simulink model "cubli_ZYX"  (R2016a)
settings: Solver=FixedStepAuto  StartTime=0.0  StopTime=10  FixedStep=0.001  RelTol=1e-3
values from neighbouring files (symbols this model uses):
  a = 0.15    [init.m]
  M = 2.5    [init.m]    (also in skew.m = [0 -z y)
  m = 0.204    [init.m]
  s = size(delta_i)    [accessibility_test.m]    (also in observability_test.m = size(delta_i,1))
  state0 = get_equilibrium(0, -pi/4, pi/2, f, state)    [init.m]
undefined symbols (not defined in the file or in its folder): X, Y, Z
libraries: sm_lib x15, nesl_utility x9
settings Model: Creator=giulio  LastModifiedBy=giulio
settings OptimizationCC: BlockReduction=off  DefaultParameterBehavior=Inlined  BufferReuse=off
settings GRTTargetCC: GeneratePreprocessorConditionals=Use local settings
settings SimscapeCC: SimscapeLogType=all  SimscapeLogDataHistory=10000

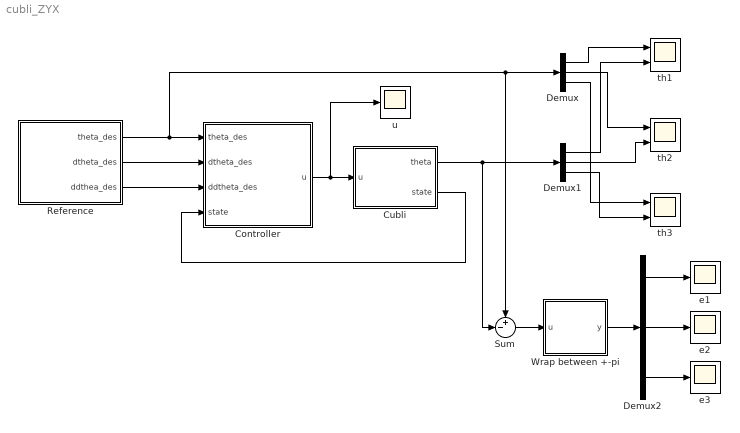
== system cubli_ZYX ==
  Controller : Subsystem
  Cubli : Subsystem
  Demux : Demux  Outputs=3
  Demux1 : Demux  Outputs=3
  Demux2 : Demux  Outputs=3
  Reference : Subsystem  mask{theta=170.0, final_time=5}
      mask prompts: final_time "Final time"
  Sum : Sum  Inputs=+-|
  Wrap between +-pi : MATLAB Function  TreatAsAtomicUnit=on
  e1 : Scope
  e2 : Scope
  e3 : Scope
  th1 : Scope  NumInputPorts=2
  th2 : Scope  NumInputPorts=2
  th3 : Scope  NumInputPorts=2
  u : Scope
  wires:
  Cubli/1(theta) -> Demux1/1, Sum/2
  Cubli/2(state) -> Controller/4(state)
  Demux/1 -> th1/1
  Demux1/1 -> th1/2
  Demux/2 -> th2/1
  Demux1/2 -> th2/2
  Demux/3 -> th3/1
  Demux1/3 -> th3/2
  Wrap between +-pi/1(y) -> Demux2/1
  Sum/1 -> Wrap between +-pi/1(u)
  Demux2/3 -> e3/1
  Demux2/1 -> e1/1
  Demux2/2 -> e2/1
  Controller/1(u) -> u/1, Cubli/1(u)
  Reference/1(theta_des) -> Controller/1(theta_des), Demux/1, Sum/1
  Reference/2(dtheta_des) -> Controller/2(dtheta_des)
  Reference/3("ddthea_des ") -> Controller/3(ddtheta_des)

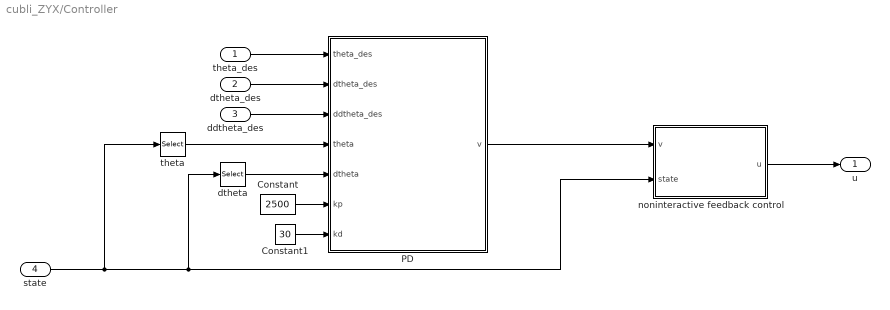
== system cubli_ZYX/Controller ==
  theta_des : Inport
  dtheta_des : Inport  Port=2
  ddtheta_des : Inport  Port=3
  state : Inport  Port=4
  Constant : Constant  Value=2500
  Constant1 : Constant  Value=30
  PD : MATLAB Function  TreatAsAtomicUnit=on
  dtheta : Selector  InputPortWidth=9  IndexOptions=Index vector (dialog)  Indices=[4 5 6]  OutputSizes=1
  noninteractive feedback control : MATLAB Function  TreatAsAtomicUnit=on
  theta : Selector  InputPortWidth=9  IndexOptions=Index vector (dialog)  Indices=[1 2 3]  OutputSizes=1
  u : Outport
  wires:
  theta_des/1 -> PD/1(theta_des)
  state/1 -> theta/1, noninteractive feedback control/2(state), dtheta/1
  PD/1(v) -> noninteractive feedback control/1(v)
  dtheta/1 -> PD/5(dtheta)
  dtheta_des/1 -> PD/2(dtheta_des)
  ddtheta_des/1 -> PD/3(ddtheta_des)
  theta/1 -> PD/4(theta)
  Constant/1 -> PD/6(kp)
  Constant1/1 -> PD/7(kd)
  noninteractive feedback control/1(u) -> u/1

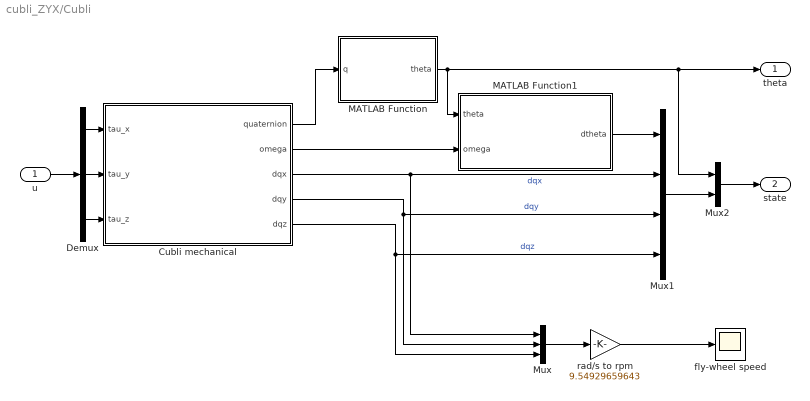
== system cubli_ZYX/Cubli ==
  u : Inport
  "Cubli mechanical " : Subsystem
  Demux : Demux  Outputs=3
  MATLAB Function : MATLAB Function  TreatAsAtomicUnit=on
  MATLAB Function1 : MATLAB Function  TreatAsAtomicUnit=on
  Mux : Mux  Inputs=3
  Mux1 : Mux
  Mux2 : Mux  Inputs=2
  fly-wheel speed : Scope
  rad/s to rpm : Gain  Gain=9.54929659643
  theta : Outport
  state : Outport  Port=2
  wires:
  Mux1/1 -> Mux2/2
  Demux/3 -> "Cubli mechanical "/3(tau_z)
  Demux/2 -> "Cubli mechanical "/2(tau_y)
  Demux/1 -> "Cubli mechanical "/1(tau_x)
  u/1 -> Demux/1
  Mux2/1 -> state/1
  "Cubli mechanical "/4(dqy) -> Mux/2, Mux1/3  "dqy"
  "Cubli mechanical "/5(dqz) -> Mux/3, Mux1/4  "dqz"
  "Cubli mechanical "/3(dqx) -> Mux/1, Mux1/2  "dqx"
  Mux/1 -> rad/s to rpm/1
  rad/s to rpm/1 -> fly-wheel speed/1
  "Cubli mechanical "/1(quaternion) -> MATLAB Function/1(q)
  MATLAB Function/1(theta) -> MATLAB Function1/1(theta), theta/1, Mux2/1
  MATLAB Function1/1(dtheta) -> Mux1/1
  "Cubli mechanical "/2(omega) -> MATLAB Function1/2(omega)

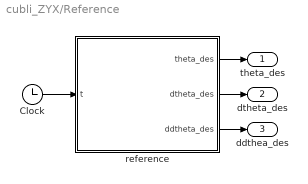
== system cubli_ZYX/Reference ==
  Clock : Clock
  reference : MATLAB Function  TreatAsAtomicUnit=on
  theta_des : Outport
  dtheta_des : Outport  Port=2
  "ddthea_des " : Outport  Port=3
  wires:
  reference/1(theta_des) -> theta_des/1
  reference/2(dtheta_des) -> dtheta_des/1
  reference/3(ddtheta_des) -> "ddthea_des "/1
  Clock/1 -> reference/1(t)

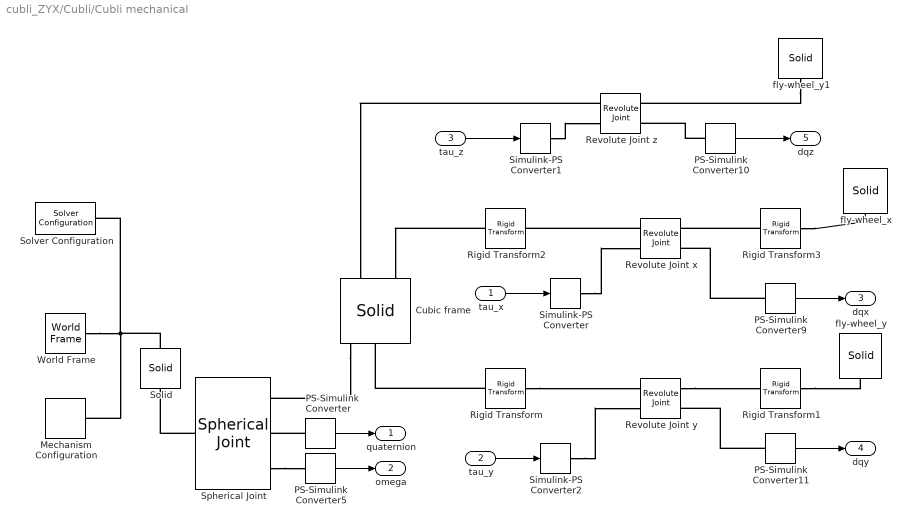
== system cubli_ZYX/Cubli/Cubli mechanical  ==
  tau_x : Inport
  tau_y : Inport  Port=2
  tau_z : Inport  Port=3
  Cubic frame : sm_lib/Body Elements/Solid  InertiaType=CalculateFromGeometry  Mass=M  MassUnits=kg  CenterOfMass=[0 0 0]  CenterOfMassUnits=m  MomentsOfInertia=[1 1 1]  MomentsOfInertiaUnits=kg*m^2  ProductsOfInertia=[0 0 0]  ProductsOfInertiaUnits=kg*m^2  DensityBased=off  Density=1000  DensityUnits=kg/(m^3)  DoExposeReferenceFrame=off  SerializedFrames=<Frames><Frame><Id>Frame1</Id><Value><Name>Oc</Name><Origin><Source>GeometricFeature</Source><FeatureName>-x -y -z point</FeatureName></Origin><PrimaryAxis><DefinedDirection>+Z</DefinedDirection><Source>ReferenceFrame</Source><SourceDirection>+Z</SourceDirection><FeatureName></FeatureName></PrimaryAxis><SecondaryAxis><DefinedDirection>+X</DefinedDirection><Source>ReferenceFrame</Source><SourceDirection>+X</SourceDirection><FeatureName></FeatureName></SecondaryAxis></Value></Frame><Frame><Id>Frame2</Id><Value><Name>Oz</Name><Origin><Source>GeometricFeature</Source><FeatureName>-z surface</FeatureName></Origin><PrimaryAxis><DefinedDirection>+Z</DefinedDirection><Source>ReferenceFrame</Source><SourceDirection>+Z</SourceDirection><FeatureName></FeatureName></PrimaryAxis><SecondaryAxis><DefinedDirection>+X</DefinedDirection><Source>ReferenceFrame</Source><SourceDirection>+X</SourceDirection><FeatureName></FeatureName></SecondaryAxis></Value></Frame><Frame><Id>Frame3</Id><Value><Name>Oy</Name><Origin><Source>GeometricFeature</Source><FeatureName>-y surface</FeatureName></Origin><PrimaryAxis><DefinedDirection>+Z</DefinedDirection><Source>ReferenceFrame</Source><SourceDirection>+Z</SourceDirection><FeatureName></FeatureName></PrimaryAxis><SecondaryAxis><DefinedDirection>+X</DefinedDirection><Source>ReferenceFrame</Source><SourceDirection>+X</SourceDirection><FeatureName></FeatureName></SecondaryAxis></Value></Frame><Frame><Id>Frame4</Id><Value><Name>Ox</Name><Origin><Source>GeometricFeature</Source><FeatureName>-x surface</FeatureName></Origin><PrimaryAxis><DefinedDirection>+Z</DefinedDirection><Source>ReferenceFrame</Source><SourceDirection>+Z</SourceDirection><FeatureName></FeatureName></PrimaryAxis><SecondaryAxis><DefinedDirection>+X</DefinedDirection><Source>ReferenceFrame</Source><SourceDirection>+X</SourceDirection><FeatureName></FeatureName></SecondaryAxis></Value></Frame><Frame><Id>Frame5</Id><Value><Name>Op</Name><Origin><Source>GeometricFeature</Source><FeatureName>+x +y +z point</FeatureName></Origin><PrimaryAxis><DefinedDirection>+Z</DefinedDirection><Source>ReferenceFrame</Source><SourceDirection>+Z</SourceDirection><FeatureName></FeatureName></PrimaryAxis><SecondaryAxis><DefinedDirection>+X</DefinedDirection><Source>ReferenceFrame</Source><SourceDirection>+X</SourceDirection><FeatureName></FeatureName></SecondaryAxis></Value></Frame></Frames>  GraphicType=FromGeometry  MarkerShape=Sphere  MarkerSize=10  GraphicVisPropType=SimpleVisualProperties  GraphicDiffuseColor=[0.5 0.5 0.5]  GraphicSpecularColor=[0.5 0.5 0.5 1.0]  GraphicAmbientColor=[0.15 0.15 0.15 1.0]  GraphicEmissiveColor=[0.0 0.0 0.0 1.0]  GraphicShininess=75  GraphicOpacity=0.9  GeometryShape=Brick  RectangleSize=[1 1]  RectangleSizeUnits=m  BrickDimensions=[a a a]  BrickDimensionUnits=m  CylinderRadius=1  CylinderRadiusUnits=m  CylinderLength=1  CylinderLengthUnits=m  SphereRadius=1  SphereRadiusUnits=m  EllipsoidRadii=[1 1 1]  EllipsoidRadiiUnits=m  ExtrusionCrossSection=[1 1; -1 1; -1 -1; 1 -1]  ExtrusionCrossSectionUnits=m  ExtrusionLength=1  ExtrusionLengthUnits=m  PolygonNumSides=3  PolygonOuterRadius=1  PolygonOuterRadiusUnits=m  ExtGeomFileType=STEP  ExtGeomFileUnits=m  RevolutionCrossSection=[1 1; 1 -1; 2 -1; 2 1]  RevolutionCrossSectionUnits=m  RevolutionExtent=Full  RevolutionAngle=180  RevolutionAngleUnits=deg
  Mechanism Configuration : sm_lib/Utilities/Mechanism Configuration  UniformGravity=Constant  GravityVector=[0 0 -9.81]  GravityUnits=m/s^2  LinearizationDelta=0.001
  PS-Simulink Converter{,5,9..11} (5 alike) : nesl_utility/PS-Simulink Converter  PhysicalDomain=network_engine_domain  SubClassName=ps_output  LeftPortType=input  RightPortType=output  PseudoPeriodic=off  Frequencies=[]  Unit=1  AffineConversion=off
  Revolute Joint x : sm_lib/Joints/Revolute Joint  SenseConstraintForce=off  SenseConstraintForceX=off  SenseConstraintForceY=off  SenseConstraintForceZ=off  SenseConstraintTorque=off  SenseConstraintTorqueX=off  SenseConstraintTorqueY=off  SenseConstraintTorqueZ=off  SenseTotalForce=off  SenseTotalForceX=off  SenseTotalForceY=off  SenseTotalForceZ=off  SenseTotalTorque=off  SenseTotalTorqueX=off  SenseTotalTorqueY=off  SenseTotalTorqueZ=off  CompositeWrenchDir=FollowerOnBase  CompositeWrenchFrame=BaseFrame  EquilibriumPosition=0  EquilibriumPositionUnits=deg  SpringStiffness=0  SpringStiffnessUnits=N*m/deg  DampingCoefficient=0  DampingCoefficientUnits=N*m/(rad/s)  TorqueActuationMode=InputTorque  MotionActuationMode=ComputedMotion  SensePosition=off  SenseVelocity=on  SenseAcceleration=off  SenseTorqueForce=off  PositionTargetSpecify=off  PositionTargetPriority=High  PositionTargetValue=0  PositionTargetValueUnits=deg  VelocityTargetSpecify=off  VelocityTargetPriority=High  VelocityTargetValue=0  VelocityTargetValueUnits=deg/s
  Revolute Joint y : sm_lib/Joints/Revolute Joint  SenseConstraintForce=off  SenseConstraintForceX=off  SenseConstraintForceY=off  SenseConstraintForceZ=off  SenseConstraintTorque=off  SenseConstraintTorqueX=off  SenseConstraintTorqueY=off  SenseConstraintTorqueZ=off  SenseTotalForce=off  SenseTotalForceX=off  SenseTotalForceY=off  SenseTotalForceZ=off  SenseTotalTorque=off  SenseTotalTorqueX=off  SenseTotalTorqueY=off  SenseTotalTorqueZ=off  CompositeWrenchDir=FollowerOnBase  CompositeWrenchFrame=BaseFrame  EquilibriumPosition=0  EquilibriumPositionUnits=deg  SpringStiffness=0  SpringStiffnessUnits=N*m/deg  DampingCoefficient=0  DampingCoefficientUnits=N*m/(rad/s)  TorqueActuationMode=InputTorque  MotionActuationMode=ComputedMotion  SensePosition=off  SenseVelocity=on  SenseAcceleration=off  SenseTorqueForce=off  PositionTargetSpecify=off  PositionTargetPriority=High  PositionTargetValue=0  PositionTargetValueUnits=deg  VelocityTargetSpecify=off  VelocityTargetPriority=High  VelocityTargetValue=0  VelocityTargetValueUnits=deg/s
  Revolute Joint z : sm_lib/Joints/Revolute Joint  SenseConstraintForce=off  SenseConstraintForceX=off  SenseConstraintForceY=off  SenseConstraintForceZ=off  SenseConstraintTorque=off  SenseConstraintTorqueX=off  SenseConstraintTorqueY=off  SenseConstraintTorqueZ=off  SenseTotalForce=off  SenseTotalForceX=off  SenseTotalForceY=off  SenseTotalForceZ=off  SenseTotalTorque=off  SenseTotalTorqueX=off  SenseTotalTorqueY=off  SenseTotalTorqueZ=off  CompositeWrenchDir=FollowerOnBase  CompositeWrenchFrame=BaseFrame  EquilibriumPosition=0  EquilibriumPositionUnits=deg  SpringStiffness=0  SpringStiffnessUnits=N*m/deg  DampingCoefficient=0  DampingCoefficientUnits=N*m/(rad/s)  TorqueActuationMode=InputTorque  MotionActuationMode=ComputedMotion  SensePosition=off  SenseVelocity=on  SenseAcceleration=off  SenseTorqueForce=off  PositionTargetSpecify=off  PositionTargetPriority=High  PositionTargetValue=0  PositionTargetValueUnits=deg  VelocityTargetSpecify=off  VelocityTargetPriority=High  VelocityTargetValue=1/6  VelocityTargetValueUnits=rev/s
  Rigid Transform : sm_lib/Frames and Transforms/Rigid Transform  TranslationMethod=None  TranslationLengthUnit=m  TranslationStandardAxis=+Z  TranslationStandardOffset=0  TranslationCartesianOffset=[0 0 0]  TranslationROffset=0  TranslationROffsetUnits=m  TranslationZOffset=0  TranslationZOffsetUnits=m  TranslationThetaOffset=0  TranslationThetaOffsetUnits=deg  RotationMethod=RotationSequence  RotationAngleUnits=deg  RotationStandardAxis=+Z  RotationAngle=0.0  RotationArbitraryAxis=[0 0 1]  FollAlignAxisA=+X  BaseAlignAxisA=+Y  FollAlignAxisB=+Y  BaseAlignAxisB=+Z  RotationSequenceAxes=FollowerAxes  RotationSequence=XYX  RotationSequenceAngles=[-90 0 0]  RotationSequenceAnglesUnits=deg  RotationMatrix=[1 0 0; 0 1 0; 0 0 1]
  Rigid Transform1 : sm_lib/Frames and Transforms/Rigid Transform  TranslationMethod=None  TranslationLengthUnit=m  TranslationStandardAxis=+Z  TranslationStandardOffset=0  TranslationCartesianOffset=[0 0 0]  TranslationROffset=0  TranslationROffsetUnits=m  TranslationZOffset=0  TranslationZOffsetUnits=m  TranslationThetaOffset=0  TranslationThetaOffsetUnits=deg  RotationMethod=RotationSequence  RotationAngleUnits=deg  RotationStandardAxis=+Z  RotationAngle=0.0  RotationArbitraryAxis=[0 0 1]  FollAlignAxisA=+X  BaseAlignAxisA=+Y  FollAlignAxisB=+Y  BaseAlignAxisB=+Z  RotationSequenceAxes=FollowerAxes  RotationSequence=XYX  RotationSequenceAngles=[90 0 0]  RotationSequenceAnglesUnits=deg  RotationMatrix=[1 0 0; 0 1 0; 0 0 1]
  Rigid Transform2 : sm_lib/Frames and Transforms/Rigid Transform  TranslationMethod=None  TranslationLengthUnit=m  TranslationStandardAxis=+Z  TranslationStandardOffset=0  TranslationCartesianOffset=[0 0 0]  TranslationROffset=0  TranslationROffsetUnits=m  TranslationZOffset=0  TranslationZOffsetUnits=m  TranslationThetaOffset=0  TranslationThetaOffsetUnits=deg  RotationMethod=RotationSequence  RotationAngleUnits=deg  RotationStandardAxis=+Z  RotationAngle=0.0  RotationArbitraryAxis=[0 0 1]  FollAlignAxisA=+X  BaseAlignAxisA=+Y  FollAlignAxisB=+Y  BaseAlignAxisB=+Z  RotationSequenceAxes=FollowerAxes  RotationSequence=XYX  RotationSequenceAngles=[0 90 0]  RotationSequenceAnglesUnits=deg  RotationMatrix=[1 0 0; 0 1 0; 0 0 1]
  Rigid Transform3 : sm_lib/Frames and Transforms/Rigid Transform  TranslationMethod=None  TranslationLengthUnit=m  TranslationStandardAxis=+Z  TranslationStandardOffset=0  TranslationCartesianOffset=[0 0 0]  TranslationROffset=0  TranslationROffsetUnits=m  TranslationZOffset=0  TranslationZOffsetUnits=m  TranslationThetaOffset=0  TranslationThetaOffsetUnits=deg  RotationMethod=RotationSequence  RotationAngleUnits=deg  RotationStandardAxis=+Z  RotationAngle=0.0  RotationArbitraryAxis=[0 0 1]  FollAlignAxisA=+X  BaseAlignAxisA=+Y  FollAlignAxisB=+Y  BaseAlignAxisB=+Z  RotationSequenceAxes=FollowerAxes  RotationSequence=XYX  RotationSequenceAngles=[0 -90 0]  RotationSequenceAnglesUnits=deg  RotationMatrix=[1 0 0; 0 1 0; 0 0 1]
  Simulink-PS Converter : nesl_utility/Simulink-PS Converter  PhysicalDomain=network_engine_domain  SubClassName=ps_input  LeftPortType=input  RightPortType=output  PseudoPeriodic=off  Frequencies=[]  NoiseDistribution=none  NoiseParameters=[]  Unit=1  AffineConversion=off  InputFiltering=off  SimscapeFilterOrder=1  InputFilterTimeConstant=0.001  UdotUserProvided=1
  Simulink-PS Converter1 : nesl_utility/Simulink-PS Converter  PhysicalDomain=network_engine_domain  SubClassName=ps_input  LeftPortType=input  RightPortType=output  PseudoPeriodic=off  Frequencies=[]  NoiseDistribution=none  NoiseParameters=[]  Unit=1  AffineConversion=off  InputFiltering=off  SimscapeFilterOrder=1  InputFilterTimeConstant=0.001  UdotUserProvided=1
  Simulink-PS Converter2 : nesl_utility/Simulink-PS Converter  PhysicalDomain=network_engine_domain  SubClassName=ps_input  LeftPortType=input  RightPortType=output  PseudoPeriodic=off  Frequencies=[]  NoiseDistribution=none  NoiseParameters=[]  Unit=1  AffineConversion=off  InputFiltering=off  SimscapeFilterOrder=1  InputFilterTimeConstant=0.001  UdotUserProvided=1
  Solid : sm_lib/Body Elements/Solid  InertiaType=CalculateFromGeometry  Mass=10^5  MassUnits=kg  CenterOfMass=[0 0 0]  CenterOfMassUnits=m  MomentsOfInertia=[1 1 1]  MomentsOfInertiaUnits=kg*m^2  ProductsOfInertia=[0 0 0]  ProductsOfInertiaUnits=kg*m^2  DensityBased=off  Density=1000  DensityUnits=kg/(m^3)  DoExposeReferenceFrame=on  SerializedFrames=<Frames><Frame><Id>Frame1</Id><Value><Name>Os</Name><Origin><Source>GeometricFeature</Source><FeatureName>+z surface</FeatureName></Origin><PrimaryAxis><DefinedDirection>+Z</DefinedDirection><Source>ReferenceFrame</Source><SourceDirection>+Z</SourceDirection><FeatureName></FeatureName></PrimaryAxis><SecondaryAxis><DefinedDirection>+X</DefinedDirection><Source>ReferenceFrame</Source><SourceDirection>+X</SourceDirection><FeatureName></FeatureName></SecondaryAxis></Value></Frame></Frames>  GraphicType=FromGeometry  MarkerShape=Sphere  MarkerSize=10  GraphicVisPropType=SimpleVisualProperties  GraphicDiffuseColor=[1.0 1.0 1.0]  GraphicSpecularColor=[0.5 0.5 0.5 1.0]  GraphicAmbientColor=[1 0.15 0.15 1.0]  GraphicEmissiveColor=[0.0 0.0 0.0 1.0]  GraphicShininess=75  GraphicOpacity=1.0  GeometryShape=Brick  RectangleSize=[1 1]  RectangleSizeUnits=m  BrickDimensions=[1 1 0.01]  BrickDimensionUnits=m  CylinderRadius=1  CylinderRadiusUnits=m  CylinderLength=1  CylinderLengthUnits=m  SphereRadius=1  SphereRadiusUnits=m  EllipsoidRadii=[1 1 1]  EllipsoidRadiiUnits=m  ExtrusionCrossSection=[1 1; -1 1; -1 -1; 1 -1]  ExtrusionCrossSectionUnits=m  ExtrusionLength=1  ExtrusionLengthUnits=m  PolygonNumSides=3  PolygonOuterRadius=1  PolygonOuterRadiusUnits=m  ExtGeomFileType=STEP  ExtGeomFileUnits=m  RevolutionCrossSection=[1 1; 1 -1; 2 -1; 2 1]  RevolutionCrossSectionUnits=m  RevolutionExtent=Full  RevolutionAngle=180  RevolutionAngleUnits=deg
  Solver Configuration : nesl_utility/Solver Configuration  PhysicalDomain=network_engine_domain  SubClassName=solver  LeftPortType=input  RightPortType=generic  Accelerate=off  Tones=[]  Harmonics=[]  SimulateNoise=off  Profile=off  UseLocalSampling=off  EnableSwitchedLinearOptims=on  FrequencyDomain=off  UseCCode=off  RelTol=0.001  AbsTol=1e-06  MinStep=1e-09  ToWorkspace=off  RevertToSquareIcSolve=off  NumHomotopyIterations=100  PhasorMode=off  PhasorModeNumHarmonics=1  OverrideAbsTol=off  DoDC=on  ResidualTolerance=1e-09  UseLocalSolver=off  LocalSolverChoice=NE_TRAPEZOIDAL_ADVANCER  LocalSolverSampleTime=0.001  DoFixedCost=off  MaxNonlinIter=3  MaxModeIter=2  LinearAlgebra=Full  DelaysMemoryBudget=1024  AutomaticFiltering=on  FilteringTimeConstant=0.001
  Spherical Joint : sm_lib/Joints/Spherical Joint  SenseConstraintForce=off  SenseConstraintForceX=off  SenseConstraintForceY=off  SenseConstraintForceZ=off  SenseConstraintTorque=off  SenseConstraintTorqueX=off  SenseConstraintTorqueY=off  SenseConstraintTorqueZ=off  SenseTotalForce=off  SenseTotalForceX=off  SenseTotalForceY=off  SenseTotalForceZ=off  SenseTotalTorque=off  SenseTotalTorqueX=off  SenseTotalTorqueY=off  SenseTotalTorqueZ=off  CompositeWrenchDir=FollowerOnBase  CompositeWrenchFrame=BaseFrame  DefPosRotationMethod=None  DefPosRotationAngleUnits=deg  DefPosRotationStandardAxis=+Z  DefPosRotationAngle=0.0  DefPosRotationArbitraryAxis=[0 0 1]  DefPosFollAlignAxisA=+X  DefPosBaseAlignAxisA=+Y  DefPosFollAlignAxisB=+Y  DefPosBaseAlignAxisB=+Z  DefPosRotationSequenceAxes=FollowerAxes  DefPosRotationSequence=XYX  DefPosRotationSequenceAngles=[0 0 0]  DefPosRotationSequenceAnglesUnits=deg  DefPosRotationMatrix=[1 0 0; 0 1 0; 0 0 1]  EqPosRotationMethod=None  EqPosRotationAngleUnits=deg  EqPosRotationStandardAxis=+Z  EqPosRotationAngle=0.0  EqPosRotationArbitraryAxis=[0 0 1]  EqPosFollAlignAxisA=+X  EqPosBaseAlignAxisA=+Y  EqPosFollAlignAxisB=+Y  EqPosBaseAlignAxisB=+Z  EqPosRotationSequenceAxes=FollowerAxes  EqPosRotationSequence=XYX  EqPosRotationSequenceAngles=[0 0 0]  EqPosRotationSequenceAnglesUnits=deg  EqPosRotationMatrix=[1 0 0; 0 1 0; 0 0 1]  SpringStiffness=0  SpringStiffnessUnits=N*m/deg  DampingCoefficient=0  DampingCoefficientUnits=N*m/(deg/s)  ActuateTorqueX=off  ActuateTorqueY=off  ActuateTorqueZ=off  ActuateTorque=off  TorqueActuationMode=NoTorque  MotionActuationMode=ComputedMotion  ActuationFrame=BaseFrame  SensePosition=on  SenseVelocityX=off  SenseVelocityY=off  SenseVelocityZ=off  SenseVelocity=on  SenseAccelerationX=off  SenseAccelerationY=off  SenseAccelerationZ=off  SenseAcceleration=off  SenseTorqueX=off  SenseTorqueY=off  SenseTorqueZ=off  SenseTorqueForce=off  SensingFrame=FollowerFrame  PositionTargetRotationMethod=RotationSequence  PositionTargetRotationAngleUnits=deg  PositionTargetRotationStandardAxis=+Z  PositionTargetRotationAngle=0.0  PositionTargetRotationArbitraryAxis=[0 0 1]  PositionTargetFollAlignAxisA=+X  PositionTargetBaseAlignAxisA=+Y  PositionTargetFollAlignAxisB=+Y  PositionTargetBaseAlignAxisB=+Z  PositionTargetRotationSequenceAxes=FollowerAxes  PositionTargetRotationSequence=ZYX  PositionTargetRotationSequenceAngles=[state0(1) state0(2) state0(3)]  PositionTargetRotationSequenceAnglesUnits=rad  PositionTargetRotationMatrix=[1 0 0; 0 1 0; 0 0 1]  PositionTargetSpecify=on  PositionTargetPriority=High  VelocityTargetValue=[0 0 0]  VelocityTargetValueUnits=deg/s  VelocityTargetSpecify=off  VelocityTargetPriority=High  VelocityTargetInFollowerFrame=on
  World Frame : sm_lib/Frames and Transforms/World Frame
  fly-wheel_x : sm_lib/Body Elements/Solid  InertiaType=CalculateFromGeometry  Mass=m  MassUnits=kg  CenterOfMass=[0 0 0]  CenterOfMassUnits=m  MomentsOfInertia=[1 1 1]  MomentsOfInertiaUnits=kg*m^2  ProductsOfInertia=[0 0 0]  ProductsOfInertiaUnits=kg*m^2  DensityBased=off  Density=1000  DensityUnits=kg/(m^3)  DoExposeReferenceFrame=off  SerializedFrames=<Frames><Frame><Id>Frame1</Id><Value><Name>Ox</Name><Origin><Source>ReferenceFrame</Source><FeatureName></FeatureName></Origin><PrimaryAxis><DefinedDirection>-X</DefinedDirection><Source>ReferenceFrame</Source><SourceDirection>+Z</SourceDirection><FeatureName></FeatureName></PrimaryAxis><SecondaryAxis><DefinedDirection>+Y</DefinedDirection><Source>ReferenceFrame</Source><SourceDirection>+X</SourceDirection><FeatureName></FeatureName></SecondaryAxis></Value></Frame></Frames>  GraphicType=FromGeometry  MarkerShape=Sphere  MarkerSize=10  GraphicVisPropType=SimpleVisualProperties  GraphicDiffuseColor=[1.0 0.0 0.0]  GraphicSpecularColor=[0.5 0.5 0.5 1.0]  GraphicAmbientColor=[0.15 0.15 0.15 1.0]  GraphicEmissiveColor=[0.0 0.0 0.0 1.0]  GraphicShininess=75  GraphicOpacity=1  GeometryShape=Cylinder  RectangleSize=[1 1]  RectangleSizeUnits=m  BrickDimensions=[a a a]  BrickDimensionUnits=m  CylinderRadius=r  CylinderRadiusUnits=m  CylinderLength=h  CylinderLengthUnits=m  SphereRadius=1  SphereRadiusUnits=m  EllipsoidRadii=[1 1 1]  EllipsoidRadiiUnits=m  ExtrusionCrossSection=[1 1; -1 1; -1 -1; 1 -1]  ExtrusionCrossSectionUnits=m  ExtrusionLength=1  ExtrusionLengthUnits=m  PolygonNumSides=3  PolygonOuterRadius=1  PolygonOuterRadiusUnits=m  ExtGeomFileType=STEP  ExtGeomFileUnits=m  RevolutionCrossSection=[1 1; 1 -1; 2 -1; 2 1]  RevolutionCrossSectionUnits=m  RevolutionExtent=Full  RevolutionAngle=180  RevolutionAngleUnits=deg
  fly-wheel_y : sm_lib/Body Elements/Solid  InertiaType=CalculateFromGeometry  Mass=m  MassUnits=kg  CenterOfMass=[0 0 0]  CenterOfMassUnits=m  MomentsOfInertia=[1 1 1]  MomentsOfInertiaUnits=kg*m^2  ProductsOfInertia=[0 0 0]  ProductsOfInertiaUnits=kg*m^2  DensityBased=off  Density=1000  DensityUnits=kg/(m^3)  DoExposeReferenceFrame=off  SerializedFrames=<Frames><Frame><Id>Frame1</Id><Value><Name>Oy</Name><Origin><Source>ReferenceFrame</Source><FeatureName></FeatureName></Origin><PrimaryAxis><DefinedDirection>+Y</DefinedDirection><Source>ReferenceFrame</Source><SourceDirection>+Z</SourceDirection><FeatureName></FeatureName></PrimaryAxis><SecondaryAxis><DefinedDirection>+X</DefinedDirection><Source>ReferenceFrame</Source><SourceDirection>+X</SourceDirection><FeatureName></FeatureName></SecondaryAxis></Value></Frame></Frames>  GraphicType=FromGeometry  MarkerShape=Sphere  MarkerSize=10  GraphicVisPropType=SimpleVisualProperties  GraphicDiffuseColor=[0.0 0.8 0.0]  GraphicSpecularColor=[0.5 0.5 0.5 1.0]  GraphicAmbientColor=[0.15 0.15 0.15 1.0]  GraphicEmissiveColor=[0.0 0.0 0.0 1.0]  GraphicShininess=75  GraphicOpacity=1  GeometryShape=Cylinder  RectangleSize=[1 1]  RectangleSizeUnits=m  BrickDimensions=[a a a]  BrickDimensionUnits=m  CylinderRadius=r  CylinderRadiusUnits=m  CylinderLength=h  CylinderLengthUnits=m  SphereRadius=1  SphereRadiusUnits=m  EllipsoidRadii=[1 1 1]  EllipsoidRadiiUnits=m  ExtrusionCrossSection=[1 1; -1 1; -1 -1; 1 -1]  ExtrusionCrossSectionUnits=m  ExtrusionLength=1  ExtrusionLengthUnits=m  PolygonNumSides=3  PolygonOuterRadius=1  PolygonOuterRadiusUnits=m  ExtGeomFileType=STEP  ExtGeomFileUnits=m  RevolutionCrossSection=[1 1; 1 -1; 2 -1; 2 1]  RevolutionCrossSectionUnits=m  RevolutionExtent=Full  RevolutionAngle=180  RevolutionAngleUnits=deg
  fly-wheel_y1 : sm_lib/Body Elements/Solid  InertiaType=CalculateFromGeometry  Mass=m  MassUnits=kg  CenterOfMass=[0 0 0]  CenterOfMassUnits=m  MomentsOfInertia=[1 1 1]  MomentsOfInertiaUnits=kg*m^2  ProductsOfInertia=[0 0 0]  ProductsOfInertiaUnits=kg*m^2  DensityBased=off  Density=1000  DensityUnits=kg/(m^3)  DoExposeReferenceFrame=off  SerializedFrames=<Frames><Frame><Id>Frame1</Id><Value><Name>Oz</Name><Origin><Source>ReferenceFrame</Source><FeatureName></FeatureName></Origin><PrimaryAxis><DefinedDirection>+Z</DefinedDirection><Source>ReferenceFrame</Source><SourceDirection>+Z</SourceDirection><FeatureName></FeatureName></PrimaryAxis><SecondaryAxis><DefinedDirection>+X</DefinedDirection><Source>ReferenceFrame</Source><SourceDirection>+X</SourceDirection><FeatureName></FeatureName></SecondaryAxis></Value></Frame></Frames>  GraphicType=FromGeometry  MarkerShape=Sphere  MarkerSize=10  GraphicVisPropType=SimpleVisualProperties  GraphicDiffuseColor=[0.0 0.0 1.0]  GraphicSpecularColor=[0.5 0.5 0.5 1.0]  GraphicAmbientColor=[0.15 0.15 0.15 1.0]  GraphicEmissiveColor=[0.0 0.0 0.0 1.0]  GraphicShininess=75  GraphicOpacity=1  GeometryShape=Cylinder  RectangleSize=[1 1]  RectangleSizeUnits=m  BrickDimensions=[a a a]  BrickDimensionUnits=m  CylinderRadius=r  CylinderRadiusUnits=m  CylinderLength=h  CylinderLengthUnits=m  SphereRadius=1  SphereRadiusUnits=m  EllipsoidRadii=[1 1 1]  EllipsoidRadiiUnits=m  ExtrusionCrossSection=[1 1; -1 1; -1 -1; 1 -1]  ExtrusionCrossSectionUnits=m  ExtrusionLength=1  ExtrusionLengthUnits=m  PolygonNumSides=3  PolygonOuterRadius=1  PolygonOuterRadiusUnits=m  ExtGeomFileType=STL  ExtGeomFileName=/home/xenvre/Downloads/flywheel/Flywheel.stl  ExtGeomFileUnits=cm  RevolutionCrossSection=[1 1; 1 -1; 2 -1; 2 1]  RevolutionCrossSectionUnits=m  RevolutionExtent=Full  RevolutionAngle=180  RevolutionAngleUnits=deg
  quaternion : Outport
  omega : Outport  Port=2
  dqx : Outport  Port=3
  dqy : Outport  Port=4
  dqz : Outport  Port=5
  wires:
  tau_y/1 -> Simulink-PS Converter2/1
  tau_z/1 -> Simulink-PS Converter1/1
  tau_x/1 -> Simulink-PS Converter/1
  PS-Simulink Converter/1 -> quaternion/1
  PS-Simulink Converter9/1 -> dqx/1
  PS-Simulink Converter10/1 -> dqz/1
  PS-Simulink Converter11/1 -> dqy/1
  PS-Simulink Converter5/1 -> omega/1
  connections:
  Rigid Transform3/LConn1 -- Revolute Joint x/RConn1
  fly-wheel_y1/LConn1 -- Revolute Joint z/RConn1
  Simulink-PS Converter2/RConn1 -- Revolute Joint y/LConn2
  Simulink-PS Converter/RConn1 -- Revolute Joint x/LConn2
  Rigid Transform1/RConn1 -- fly-wheel_y/LConn1
  Cubic frame/LConn1 -- Spherical Joint/RConn1
  World Frame/RConn1 -- Solid/RConn1 -- Solver Configuration/RConn1 -- Mechanism Configuration/RConn1
  Simulink-PS Converter1/RConn1 -- Revolute Joint z/LConn2
  Revolute Joint y/RConn1 -- Rigid Transform1/LConn1
  Revolute Joint x/LConn1 -- Rigid Transform2/RConn1
  Rigid Transform/RConn1 -- Revolute Joint y/LConn1
  PS-Simulink Converter/LConn1 -- Spherical Joint/RConn2
  PS-Simulink Converter9/LConn1 -- Revolute Joint x/RConn2
  PS-Simulink Converter10/LConn1 -- Revolute Joint z/RConn2
  PS-Simulink Converter11/LConn1 -- Revolute Joint y/RConn2
  Rigid Transform2/LConn1 -- Cubic frame/RConn2
  Revolute Joint z/LConn1 -- Cubic frame/RConn1
  Rigid Transform/LConn1 -- Cubic frame/LConn2
  Rigid Transform3/RConn1 -- fly-wheel_x/LConn1
  Spherical Joint/LConn1 -- Solid/LConn1
  Spherical Joint/RConn3 -- PS-Simulink Converter5/LConn1

== matlab function cubli_ZYX/Controller/PD ==
  data: theta_des input; dtheta_des input; ddtheta_des input; theta input; v output; dtheta input; kp input; kd input
function v = fcn(theta_des,dtheta_des,ddtheta_des, theta, dtheta, kp, kd)
coder.extrinsic('wrapToPi');

error = zeros(3,1);

%  wrap the angle bewteen -pi and +pi
error = wrapToPi(theta_des - theta);

Kp = kp * eye(3);
Kd = kd * eye(3);

v = Kp * error + Kd * (dtheta_des - dtheta) + ddtheta_des;

== matlab function cubli_ZYX/Controller/noninteractive feedback control ==
  data: v input; state input; u output
  function u = nic_fnc(v, state)

th1 = state(1);
th2 = state(2);
th3 = state(3);

th1dot = state(4);
th2dot = state(5);
th3dot = state(6);
qxdot = state(7);
qydot = state(8);
qzdot = state(9);


A = [                                                                   -(1123197656438253912603716965936891166720000*2^(1/2)*sin(th3 + pi/4))/(50688073959935957106266099682798465939237*cos(th2)),                                                    -(11529215046068469760000*(97421867139278569472*cos(th3) + 173808361171031714041*sin(th3)))/(50688073959935957106266099682798465939237*cos(th2)),                                                    -(11529215046068469760000*(173808361171031714041*cos(th3) + 97421867139278569472*sin(th3)))/(50688073959935957106266099682798465939237*cos(th2))
                                                                                   -(1123197656438253912603716965936891166720000*2^(1/2)*cos(th3 + pi/4))/50688073959935957106266099682798465939237, (1123197656438253912603716965936891166720000*sin(th3))/50688073959935957106266099682798465939237 - (2003873972745561633640040521298775900160000*cos(th3))/50688073959935957106266099682798465939237, (2003873972745561633640040521298775900160000*sin(th3))/50688073959935957106266099682798465939237 - (1123197656438253912603716965936891166720000*cos(th3))/50688073959935957106266099682798465939237
 -(11529215046068469760000*(173808361171031714041*cos(th2) + 97421867139278569472*cos(th3)*sin(th2) + 97421867139278569472*sin(th2)*sin(th3)))/(50688073959935957106266099682798465939237*cos(th2)),  -(11529215046068469760000*(97421867139278569472*cos(th2) + 97421867139278569472*cos(th3)*sin(th2) + 173808361171031714041*sin(th2)*sin(th3)))/(50688073959935957106266099682798465939237*cos(th2)),  -(11529215046068469760000*(97421867139278569472*cos(th2) + 173808361171031714041*cos(th3)*sin(th2) + 97421867139278569472*sin(th2)*sin(th3)))/(50688073959935957106266099682798465939237*cos(th2))];
 

b = [                                                                                                                                                                                                                                                                                                                                                                                                                                                                                                                                                                                                                                                                                                                                                                                                                                                                                                                                                                                                                                                                                                                                                                                                                                                                                                                                                                                                (37208574363983751213784670214039629987840*th1dot^2*cos(th3) - 37208574363983751213784670214039629987840*th2dot^2*cos(th3) + 37208574363983751213784670214039629987840*th3dot^2*cos(th3) - 37208574363983751213784670214039629987840*th1dot^2*sin(th3) + 37208574363983751213784670214039629987840*th2dot^2*sin(th3) - 37208574363983751213784670214039629987840*th3dot^2*sin(th3) - 5234057499985498930356104062315637394898944*cos(th3)*sin(th2) + 5234057499985498930356104062315637394898944*sin(th2)*sin(th3) + 1419410730694772925795933922925238500000*qxdot*th2dot - 795598339977096578581794905915392000000*qydot*th2dot + 140800205444266547517405832452217960942325*th2dot*th3dot + 18604287181991875606892335107019814993920*th1dot^2*sin(2*th2) + 795598339977096578581794905915392000000*qxdot*th1dot*cos(th2) - 1419410730694772925795933922925238500000*qydot*th3dot*cos(th3) - 795598339977096578581794905915392000000*qzdot*th1dot*cos(th2) + 795598339977096578581794905915392000000*qzdot*th3dot*cos(th3) - 37208574363983751213784670214039629987840*th1dot*th3dot*cos(th2) - 795598339977096578581794905915392000000*qydot*th3dot*sin(th3) + 1419410730694772925795933922925238500000*qzdot*th3dot*sin(th3) + 140800205444266547517405832452217960942325*th1dot*th2dot*sin(th2) - 37208574363983751213784670214039629987840*th1dot^2*cos(th2)^2*cos(th3) + 37208574363983751213784670214039629987840*th1dot^2*cos(th2)^2*sin(th3) + 795598339977096578581794905915392000000*qydot*th2dot*cos(th3)^2 - 795598339977096578581794905915392000000*qzdot*th2dot*cos(th3)^2 + 795598339977096578581794905915392000000*qxdot*th2dot*sin(2*th3) - 397799169988548289290897452957696000000*qydot*th2dot*sin(2*th3) - 397799169988548289290897452957696000000*qzdot*th2dot*sin(2*th3) - 37208574363983751213784670214039629987840*th2dot*th3dot*sin(2*th3) + 1419410730694772925795933922925238500000*qydot*th1dot*cos(th3)*sin(th2) - 795598339977096578581794905915392000000*qzdot*th1dot*cos(th3)*sin(th2) - 37208574363983751213784670214039629987840*th1dot*th2dot*cos(th2)*sin(th3) - 74417148727967502427569340428079259975680*th1dot*th3dot*cos(th3)*sin(th2) + 795598339977096578581794905915392000000*qydot*th1dot*sin(th2)*sin(th3) - 1419410730694772925795933922925238500000*qzdot*th1dot*sin(th2)*sin(th3) + 74417148727967502427569340428079259975680*th1dot*th3dot*sin(th2)*sin(th3) - 74417148727967502427569340428079259975680*th1dot^2*cos(th2)*cos(th3)^2*sin(th2) - 1591196679954193157163589811830784000000*qxdot*th1dot*cos(th2)*cos(th3)^2 + 795598339977096578581794905915392000000*qydot*th1dot*cos(th2)*cos(th3)^2 + 795598339977096578581794905915392000000*qzdot*th1dot*cos(th2)*cos(th3)^2 + 74417148727967502427569340428079259975680*th1dot*th3dot*cos(th2)*cos(th3)^2 - 37208574363983751213784670214039629987840*th1dot*th2dot*cos(th2)*cos(th3) + 795598339977096578581794905915392000000*qydot*th1dot*cos(th2)*cos(th3)*sin(th3) - 795598339977096578581794905915392000000*qzdot*th1dot*cos(th2)*cos(th3)*sin(th3) + 74417148727967502427569340428079259975680*th1dot*th2dot*cos(th3)*sin(th2)*sin(th3))/(140800205444266547517405832452217960942325*cos(th2))
                                                                                                                                                                                                                                                                                                                                                                                                                                                                                                                                                                                             (68520719092170281189376*cos(th2))/1843260477247944264925 - (97421867139278569472*th1dot^2*cos(th3))/368652095449588852985 - (97421867139278569472*th3dot^2*cos(th3))/368652095449588852985 - (97421867139278569472*th1dot^2*sin(th3))/368652095449588852985 - (97421867139278569472*th3dot^2*sin(th3))/368652095449588852985 + (68520719092170281189376*cos(th3)*sin(th2))/1843260477247944264925 + (68520719092170281189376*sin(th2)*sin(th3))/1843260477247944264925 - (31823933599083863143271796236615680000*qxdot*th2dot)/5632008217770661900696233298088718437693 + (31823933599083863143271796236615680000*qydot*th2dot)/5632008217770661900696233298088718437693 + (97421867139278569472*th2dot*th3dot)/368652095449588852985 - (56776429227790917031837356917009540000*qxdot*th1dot*cos(th2))/5632008217770661900696233298088718437693 - (31823933599083863143271796236615680000*qydot*th3dot*cos(th3))/5632008217770661900696233298088718437693 + (31823933599083863143271796236615680000*qzdot*th1dot*cos(th2))/5632008217770661900696233298088718437693 + (56776429227790917031837356917009540000*qzdot*th3dot*cos(th3))/5632008217770661900696233298088718437693 - th1dot*th3dot*cos(th2) + (56776429227790917031837356917009540000*qydot*th3dot*sin(th3))/5632008217770661900696233298088718437693 - (31823933599083863143271796236615680000*qzdot*th3dot*sin(th3))/5632008217770661900696233298088718437693 - (97421867139278569472*th1dot*th2dot*sin(th2))/368652095449588852985 + (194843734278557138944*th1dot^2*cos(th2)^2*cos(th3))/368652095449588852985 + (194843734278557138944*th1dot^2*cos(th2)^2*sin(th3))/368652095449588852985 + (63647867198167726286543592473231360000*qxdot*th2dot*cos(th3)^2)/5632008217770661900696233298088718437693 - (31823933599083863143271796236615680000*qydot*th2dot*cos(th3)^2)/5632008217770661900696233298088718437693 - (31823933599083863143271796236615680000*qzdot*th2dot*cos(th3)^2)/5632008217770661900696233298088718437693 - (194843734278557138944*th2dot*th3dot*cos(th3)^2)/368652095449588852985 - (15911966799541931571635898118307840000*qydot*th2dot*sin(2*th3))/5632008217770661900696233298088718437693 + (15911966799541931571635898118307840000*qzdot*th2dot*sin(2*th3))/5632008217770661900696233298088718437693 + (31823933599083863143271796236615680000*qydot*th1dot*cos(th3)*sin(th2))/5632008217770661900696233298088718437693 - (56776429227790917031837356917009540000*qzdot*th1dot*cos(th3)*sin(th2))/5632008217770661900696233298088718437693 - (97421867139278569472*th1dot*th2dot*cos(th2)*sin(th3))/368652095449588852985 + (194843734278557138944*th1dot*th3dot*cos(th3)*sin(th2))/368652095449588852985 - (56776429227790917031837356917009540000*qydot*th1dot*sin(th2)*sin(th3))/5632008217770661900696233298088718437693 + (31823933599083863143271796236615680000*qzdot*th1dot*sin(th2)*sin(th3))/5632008217770661900696233298088718437693 + (194843734278557138944*th1dot*th3dot*sin(th2)*sin(th3))/368652095449588852985 + (31823933599083863143271796236615680000*qydot*th1dot*cos(th2)*cos(th3)^2)/5632008217770661900696233298088718437693 - (31823933599083863143271796236615680000*qzdot*th1dot*cos(th2)*cos(th3)^2)/5632008217770661900696233298088718437693 + (194843734278557138944*th1dot*th2dot*cos(th3)^2*sin(th2))/368652095449588852985 + (97421867139278569472*th1dot*th2dot*cos(th2)*cos(th3))/368652095449588852985 + (194843734278557138944*th1dot^2*cos(th2)*cos(th3)*sin(th2)*sin(th3))/368652095449588852985 + (63647867198167726286543592473231360000*qxdot*th1dot*cos(th2)*cos(th3)*sin(th3))/5632008217770661900696233298088718437693 - (31823933599083863143271796236615680000*qydot*th1dot*cos(th2)*cos(th3)*sin(th3))/5632008217770661900696233298088718437693 - (31823933599083863143271796236615680000*qzdot*th1dot*cos(th2)*cos(th3)*sin(th3))/5632008217770661900696233298088718437693 - (194843734278557138944*th1dot*th3dot*cos(th2)*cos(th3)*sin(th3))/368652095449588852985
 (5234057499985498930356104062315637394898944*sin(th3) - 5234057499985498930356104062315637394898944*cos(th3) + 37208574363983751213784670214039629987840*th1dot^2*cos(th2) - 37208574363983751213784670214039629987840*th2dot^2*cos(th2) + 140800205444266547517405832452217960942325*th1dot*th2dot - 37208574363983751213784670214039629987840*th1dot^2*sin(th2)*sin(th3) + 37208574363983751213784670214039629987840*th2dot^2*sin(th2)*sin(th3) - 37208574363983751213784670214039629987840*th3dot^2*sin(th2)*sin(th3) + 1419410730694772925795933922925238500000*qydot*th1dot*cos(th3) - 795598339977096578581794905915392000000*qydot*th3dot*cos(th2) - 795598339977096578581794905915392000000*qzdot*th1dot*cos(th3) + 795598339977096578581794905915392000000*qzdot*th3dot*cos(th2) - 74417148727967502427569340428079259975680*th1dot*th3dot*cos(th3) + 1419410730694772925795933922925238500000*qxdot*th2dot*sin(th2) + 795598339977096578581794905915392000000*qydot*th1dot*sin(th3) - 795598339977096578581794905915392000000*qydot*th2dot*sin(th2) - 1419410730694772925795933922925238500000*qzdot*th1dot*sin(th3) + 74417148727967502427569340428079259975680*th1dot*th3dot*sin(th3) + 140800205444266547517405832452217960942325*th2dot*th3dot*sin(th2) - 74417148727967502427569340428079259975680*th1dot^2*cos(th2)*cos(th3)^2 + 74417148727967502427569340428079259975680*th2dot^2*cos(th2)*cos(th3)^2 + 397799169988548289290897452957696000000*qxdot*th1dot*sin(2*th2) + 397799169988548289290897452957696000000*qydot*th1dot*sin(2*th2) - 795598339977096578581794905915392000000*qzdot*th1dot*sin(2*th2) + 37208574363983751213784670214039629987840*th1dot*th2dot*sin(2*th3) - 18604287181991875606892335107019814993920*th1dot*th3dot*sin(2*th2) + 37208574363983751213784670214039629987840*th1dot^2*cos(th3)*sin(th2) - 37208574363983751213784670214039629987840*th2dot^2*cos(th3)*sin(th2) + 37208574363983751213784670214039629987840*th3dot^2*cos(th3)*sin(th2) + 795598339977096578581794905915392000000*qxdot*th2dot*cos(th2)*sin(th3) - 1419410730694772925795933922925238500000*qydot*th2dot*cos(th2)*sin(th3) - 1419410730694772925795933922925238500000*qydot*th3dot*cos(th3)*sin(th2) + 795598339977096578581794905915392000000*qzdot*th3dot*cos(th3)*sin(th2) + 37208574363983751213784670214039629987840*th2dot*th3dot*cos(th2)*sin(th3) - 795598339977096578581794905915392000000*qydot*th3dot*sin(th2)*sin(th3) + 1419410730694772925795933922925238500000*qzdot*th3dot*sin(th2)*sin(th3) - 795598339977096578581794905915392000000*qxdot*th1dot*cos(th2)^2*cos(th3) + 795598339977096578581794905915392000000*qzdot*th1dot*cos(th2)^2*cos(th3) + 37208574363983751213784670214039629987840*th1dot*th3dot*cos(th2)^2*cos(th3) + 795598339977096578581794905915392000000*qxdot*th1dot*cos(th2)^2*sin(th3) - 795598339977096578581794905915392000000*qydot*th1dot*cos(th2)^2*sin(th3) + 795598339977096578581794905915392000000*qydot*th2dot*cos(th3)^2*sin(th2) - 795598339977096578581794905915392000000*qzdot*th2dot*cos(th3)^2*sin(th2) - 37208574363983751213784670214039629987840*th1dot*th3dot*cos(th2)^2*sin(th3) + 795598339977096578581794905915392000000*qxdot*th2dot*cos(th2)*cos(th3) - 1419410730694772925795933922925238500000*qzdot*th2dot*cos(th2)*cos(th3) + 37208574363983751213784670214039629987840*th2dot*th3dot*cos(th2)*cos(th3) - 1591196679954193157163589811830784000000*qxdot*th1dot*cos(th2)*cos(th3)^2*sin(th2) + 795598339977096578581794905915392000000*qydot*th1dot*cos(th2)*cos(th3)^2*sin(th2) + 795598339977096578581794905915392000000*qzdot*th1dot*cos(th2)*cos(th3)^2*sin(th2) + 74417148727967502427569340428079259975680*th1dot*th2dot*cos(th2)^2*cos(th3)*sin(th3) + 74417148727967502427569340428079259975680*th1dot*th3dot*cos(th2)*cos(th3)^2*sin(th2) - 74417148727967502427569340428079259975680*th1dot*th2dot*cos(th2)*cos(th3)*sin(th2) + 1591196679954193157163589811830784000000*qxdot*th2dot*cos(th3)*sin(th2)*sin(th3) - 795598339977096578581794905915392000000*qydot*th2dot*cos(th3)*sin(th2)*sin(th3) - 795598339977096578581794905915392000000*qzdot*th2dot*cos(th3)*sin(th2)*sin(th3) - 74417148727967502427569340428079259975680*th1dot*th2dot*cos(th2)*sin(th2)*sin(th3) - 74417148727967502427569340428079259975680*th2dot*th3dot*cos(th3)*sin(th2)*sin(th3) + 795598339977096578581794905915392000000*qydot*th1dot*cos(th2)*cos(th3)*sin(th2)*sin(th3) - 795598339977096578581794905915392000000*qzdot*th1dot*cos(th2)*cos(th3)*sin(th2)*sin(th3))/(140800205444266547517405832452217960942325*cos(th2))];


u = -A \ b + A \ v;
end

== matlab function cubli_ZYX/Cubli/MATLAB Function ==
  data: q input; theta output
function theta = quat_to_euler(q)
%#codegen
theta = quat2eul(q');

== matlab function cubli_ZYX/Cubli/MATLAB Function1 ==
  data: theta input; omega input; dtheta output
function dtheta = omega_to_dtheta(theta, omega)
th2 = theta(2);
th3 = theta(3);

dtheta = [0, sin(th3)/cos(th2), cos(th3)/cos(th2)
           0, cos(th3), -sin(th3)
           1, (sin(th2)*sin(th3))/cos(th2), (cos(th3)*sin(th2))/cos(th2)]*omega;

== matlab function cubli_ZYX/Reference/reference ==
  data: t input; theta_des output; dtheta_des output; ddtheta_des output; state0 parameter; final_time parameter; theta parameter
function [theta_des, dtheta_des, ddtheta_des] = reference(t, state0, final_time, theta)

coder.extrinsic('wrapToPi');

theta = theta * pi / 180;

th1 = state0(1);
th2 = state0(2);
th3 = state0(3);

state_0 = [th1;th2;th3];
state_f = state_0 + theta * [1;0;0];
state_f = wrapToPi(state_f);

a0 = state_0;
a1 = [0;0;0];
a2 = [0;0;0];

a3 = 10/(final_time^3) * (state_f - state_0);
a4 = -15/(final_time^4) * (state_f - state_0);
a5 = 6/(final_time^5) * (state_f - state_0);

if t>final_time
    t = final_time;
end

theta_des = a5 * t^5 + a4 * t^4 + a3 * t^3 + a2 * t^2 + a1 * t + a0;
dtheta_des = 5 * a5 * t^4 + 4 * a4 * t^3 + 3 * a3 * t^2  + 2 * a2 * t + a1;
ddtheta_des = 5 * 4 * a5 * t^3 + 4 * 3 * a4 * t^2 + 3 * 2 * a3 * t + 2 * a2;

end

== matlab function cubli_ZYX/Wrap between +-pi ==
  data: u input; y output
function y = wrap(u)
coder.extrinsic('wrapToPi');

y = [0;0;0];
y = wrapToPi(u);
